simulink model "wheelSpeedSystem0"  (R2021a)
settings: Solver=VariableStepAuto  StartTime=0.0  StopTime=10.0  RelTol=1e-3
undefined symbols (not defined in the file): I, Kf, PBmax, Rr, TB, v0
settings Model: Creator=Utkarsh Anand  LastModifiedBy=Utkarsh Anand
settings DataIOCC: SaveOutput=off  SaveTime=off

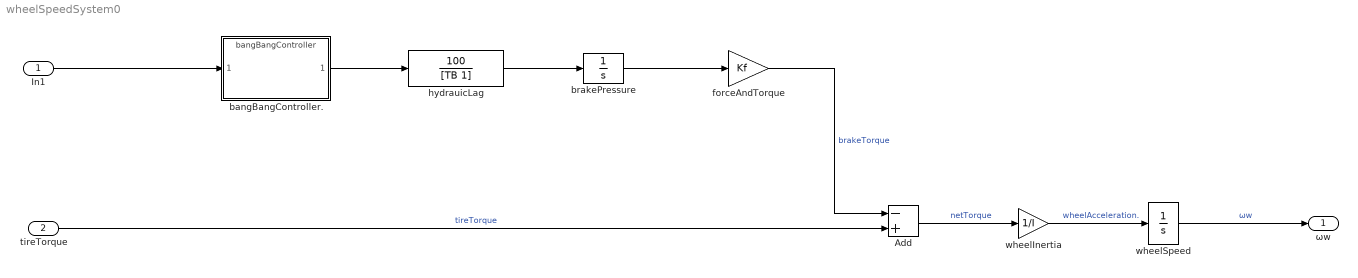
== system wheelSpeedSystem0 ==
  In1 : Inport  OutDataTypeStr=double  PortDimensions=1  SampleTime=0
  tireTorque : Inport  Port=2  OutDataTypeStr=double  PortDimensions=1  SampleTime=0
  Add : Sum  Inputs=-+
  bangBangController. : ModelReference  ModelNameDialog=bangBangController  SimulationMode=Normal  ModelReferenceVersion=1.27
  brakePressure : Integrator  LimitOutput=on  UpperSaturationLimit=PBmax  LowerSaturationLimit=0
  forceAndTorque : Gain  Gain=Kf  SaturateOnIntegerOverflow=on  OutDataTypeStr=Inherit: Same as input  ParamDataTypeStr=Inherit: Same as input
  hydrauicLag : TransferFcn  Numerator=[100]  Denominator=[TB 1]
  wheelInertia : Gain  Gain=1/I
  wheelSpeed : Integrator  InitialCondition=v0/Rr  LimitOutput=on  UpperSaturationLimit=1000  LowerSaturationLimit=0
  ωw : Outport  OutDataTypeStr=double  PortDimensions=1  SampleTime=0
  wires:
  In1/1 -> bangBangController./1
  hydrauicLag/1 -> brakePressure/1
  brakePressure/1 -> forceAndTorque/1
  Add/1 -> wheelInertia/1  "netTorque"
  wheelInertia/1 -> wheelSpeed/1  "wheelAcceleration."
  bangBangController./1 -> hydrauicLag/1
  forceAndTorque/1 -> Add/1  "brakeTorque"
  tireTorque/1 -> Add/2  "tireTorque"
  wheelSpeed/1 -> ωw/1  "ωw"
